simulink model "tv_remote_ass"  (R2020a)
settings: Solver=VariableStepAuto  StartTime=0.0  StopTime=10.0  RelTol=1e-3
settings Model: Creator=Ujwal  LastModifiedBy=Ujwal

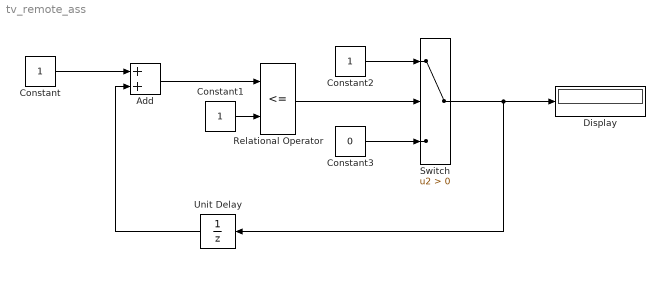
== system tv_remote_ass ==
  Add : Sum
  Constant : Constant
  Constant1 : Constant
  Constant2 : Constant
  Constant3 : Constant  Value=0
  Display : Display
  Relational Operator : RelationalOperator  Operator=<=  OutDataTypeStr=boolean  RndMeth=Simplest
  Switch : Switch  Criteria=u2 > Threshold
  Unit Delay : UnitDelay  SampleTime=-1  HasFrameUpgradeWarning=on
  wires:
  Constant/1 -> Add/1
  Constant1/1 -> Relational Operator/2
  Add/1 -> Relational Operator/1
  Relational Operator/1 -> Switch/2
  Unit Delay/1 -> Add/2
  Switch/1 -> Unit Delay/1, Display/1
  Constant3/1 -> Switch/3
  Constant2/1 -> Switch/1
